simulink model "power_13NodeTestFeeder_4VSC_PV_DEG_symmtrc_loads_"  (R2024b)
settings: Solver=ode15s  StartTime=0.0  StopTime=5  FixedStep=1e-6  MaxStep=1e-4  RelTol=1e-6  AbsTol=1e-8  EnableMultiTasking=on
PreLoadFcn:
  | %power_13NodeTestFeeder_init;
values from neighbouring files (symbols this model uses):
  a = 1.3    [init_para_with_symmtrc_loads.m]
  Cdc = 278e-3    (= 0.278)    [init_para_with_symmtrc_loads.m]
  fg = 60    [a01_scan_VSC_13_feeder.m]    (also in init_para_with_symmtrc_loads.m)
  Gn = 1000    [init_para_with_symmtrc_loads.m]
  H = 8    [init_para_with_symmtrc_loads.m]
  Ipv_n = Isc_n*(Rp+Rs)/Rp    (= 8.21426513558)    [init_para_with_symmtrc_loads.m]
  Isc_n = 8.21    [init_para_with_symmtrc_loads.m]
  k = 1.3806503e-23    [init_para_with_symmtrc_loads.m]    (also in ypm_plot_compare_ana_meas.m = 2)
  Kdroop = Sn/(Rdroop*60)    (= 4166666.66667)    [init_para_with_symmtrc_loads.m]
  KI = 0.0032    [init_para_with_symmtrc_loads.m]
  Ki_C = Rc/tau_C    (= 0.768)    [init_para_with_symmtrc_loads.m]
  Ki_DC = omega_DC^2*Cdc    [init_para_with_symmtrc_loads.m]
  ki_dvpp = kp_dvpp/Ti_dvpp    [init_para_with_symmtrc_loads.m]
  Ki_P = 1/(Ki_pq*tau_P)    [init_para_with_symmtrc_loads.m]
  Ki_PLL = Kp_PLL/tau_PLL    [init_para_with_symmtrc_loads.m]
  Kp_C = Lc/tau_C    (= 0.020372)    [init_para_with_symmtrc_loads.m]
  Kp_DC = 2*xi_DC*omega_DC*Cdc    [init_para_with_symmtrc_loads.m]
  kp_dvpp = -(2*Kdcgain)^-1    [init_para_with_symmtrc_loads.m]
  Kp_P = tau_C/(Ki_pq*tau_P)    [init_para_with_symmtrc_loads.m]
  Kp_PLL = xi_PLL*2*omega_PLL/Vp    [init_para_with_symmtrc_loads.m]
  KV = -0.123    [init_para_with_symmtrc_loads.m]
  kv_Vp = [ 1.021 1.042 1.0174]    [init_para_with_symmtrc_loads.m]
  KVmp = Vmp_n/Voc_n    (= 0.799392097264)    [init_para_with_symmtrc_loads.m]
  Lc = 20.372e-6    (= 2.0372e-05)    [init_para_with_symmtrc_loads.m]
  Lg = Xg /(2*pi*fg)    [init_para_with_symmtrc_loads.m]
  Np = 345    [init_para_with_symmtrc_loads.m]
  Ns = 45    [init_para_with_symmtrc_loads.m]
  Ns_cell = 54    [init_para_with_symmtrc_loads.m]
  p_jump_time = 5    [init_para_with_symmtrc_loads.m]
  p_jump_value = 2*-1e6    (= -2000000)    [init_para_with_symmtrc_loads.m]
  phi_vec = phi_vec_deg/180*pi    [init_para_with_symmtrc_loads.m]
  ppv_nom = 4.9687e+05    (= 496870)    [init_para_with_symmtrc_loads.m]
  q = 1.6021764e-19    [init_para_with_symmtrc_loads.m]
  Rc = 0.768e-3    (= 0.000768)    [init_para_with_symmtrc_loads.m]
  Rg = (U_rms^2 / S_sc) / (sqrt(1 + XoverR^2))    [init_para_with_symmtrc_loads.m]
  Rp = 425.405    [init_para_with_symmtrc_loads.m]
  Rs = 0.221    [init_para_with_symmtrc_loads.m]
  S_base_all = 1    [init_para_with_symmtrc_loads.m]
  Sn = 15e6    (= 15000000)    [init_para_with_symmtrc_loads.m]
  tau_PLL = 2*xi_PLL/omega_PLL    [init_para_with_symmtrc_loads.m]
  Tn = 25    [init_para_with_symmtrc_loads.m]
  Ts = T_ctrl/n_ctrl    [a01_scan_VSC_13_feeder.m]    (also in init_para_with_symmtrc_loads.m = 5e-05)
  U_rms = 4160    [init_para_with_symmtrc_loads.m]
  Vdc = 1200    [init_para_with_symmtrc_loads.m]
  Voc_n = 32.9    [init_para_with_symmtrc_loads.m]
  Vp = sqrt(2)*480/sqrt(3)    [a01_scan_VSC_13_feeder.m]    (also in init_para_with_symmtrc_loads.m = Ug*sqrt(2)/sqrt(3))
undefined symbols (not defined in the file or in its folder): j, Newton, para_grid, para_PVgeno, Raphson
libraries: spsabctoAlphaBetaZeroLib x141, spsPower3phInstantaneousLib x70, spsSeriesRLCBranchLib x44, spsThreePhaseVIMeasurementLib x27, slpidlib x24, spsThreePhaseSeriesRLCLoadLib x15, spsControlledVoltageSourceLib x15, spsMeanLib x9, spsCurrentMeasurementLib x8, spsControlledCurrentSourceLib x8, cstblocks x8, spsGroundLib x5
(part 7 of 10)

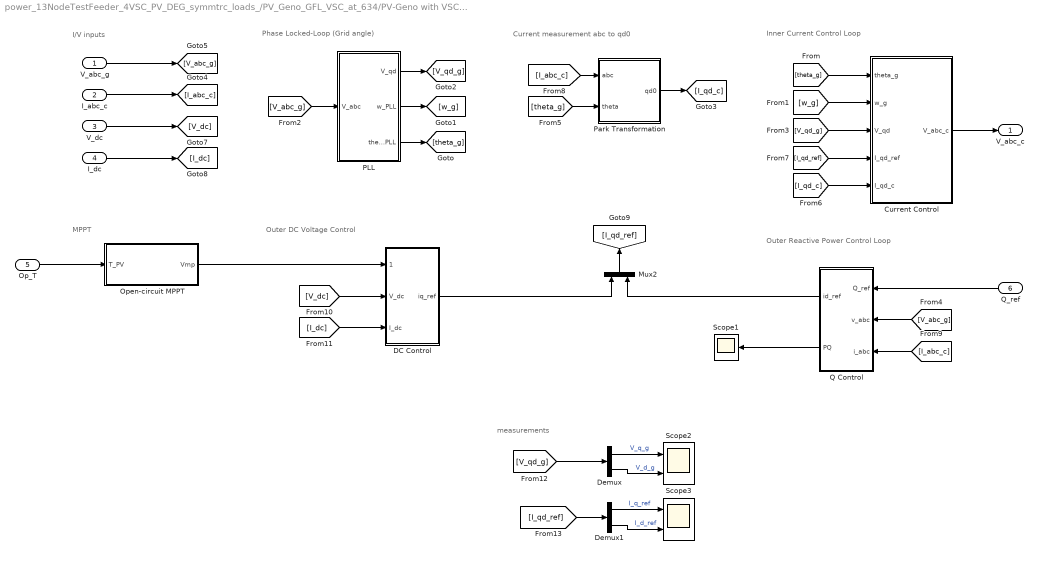
== system power_13NodeTestFeeder_4VSC_PV_DEG_symmtrc_loads_/PV_Geno_GFL_VSC_at_634/PV-Geno with VSC_GFL_at_634     /VSC Control ==
  note: I/V inputs
  note: Phase Locked-Loop (Grid angle)
  note: Current measurement abc to qd0
  note: Inner Current Control Loop
  note: Outer Reactive Power Control Loop
  note: MPPT
  note: Outer DC Voltage Control
  note: measurements
  V_abc_g : Inport
  I_abc_c : Inport  Port=2
  V_dc : Inport  Port=3
  I_dc : Inport  Port=4
  Op_T : Inport  Port=5
  Q_ref : Inport  Port=6
  Current Control : Subsystem
  DC Control : Subsystem
  Demux : Demux  Outputs=2
  Demux1 : Demux  Outputs=2
  Mux2 : Mux  Inputs=2
  Open-circuit MPPT : Subsystem
  PLL : Subsystem
  Park Transformation : Subsystem
  Q Control : Subsystem
  Scope1 : Scope
  Scope2 : Scope  NumInputPorts=2
  Scope3 : Scope  NumInputPorts=2
  V_abc_c : Outport
  wires:
  Park Transformation/1(qd0) -> [I_qd_c]
  [theta_g] -> Current Control/1(theta_g)
  PLL/3(theta_PLL) -> [theta_g]
  [I_qd_ref] -> Current Control/4(I_qd_ref)
  [theta_g] -> Park Transformation/2(theta)
  PLL/1(V_qd) -> [V_qd_g]
  PLL/2(w_PLL) -> [w_g]
  [w_g] -> Current Control/2(w_g)
  [V_qd_g] -> Current Control/3(V_qd)
  [I_qd_c] -> Current Control/5(I_qd_c)
  Current Control/1(V_abc_c) -> V_abc_c/1
  [V_abc_g] -> Q Control/2(v_abc)
  [I_abc_c] -> Q Control/3(i_abc)
  [V_dc] -> DC Control/2(V_dc)
  [I_dc] -> DC Control/3(I_dc)
  [I_abc_c] -> Park Transformation/1(abc)
  V_dc/1 -> [V_dc]
  I_abc_c/1 -> [I_abc_c]
  V_abc_g/1 -> [V_abc_g]
  I_dc/1 -> [I_dc]
  DC Control/1(iq_ref) -> Mux2/1
  Q Control/1(id_ref) -> Mux2/2
  Mux2/1 -> [I_qd_ref]
  Q_ref/1 -> Q Control/1(Q_ref)
  Op_T/1 -> Open-circuit MPPT/1(T_PV)
  Q Control/2(PQ) -> Scope1/1
  Open-circuit MPPT/1(Vmp) -> DC Control/1(V_dc_ref)
  [V_abc_g] -> PLL/1(V_abc)
  Demux/2 -> Scope2/2  "V_d_g"
  Demux1/2 -> Scope3/2  "I_d_ref"
  Demux/1 -> Scope2/1  "V_q_g"
  [V_qd_g] -> Demux/1
  Demux1/1 -> Scope3/1  "I_q_ref"
  [I_qd_ref] -> Demux1/1

== system power_13NodeTestFeeder_4VSC_PV_DEG_symmtrc_loads_/PV_Geno_GFL_VSC_at_672/PV-Geno with VSC_GFL_at_672/PV Array ==
  note: Allows PV model to initialize
  T : Inport
  G : Inport  Port=2
  V_dc : Inport  Port=3
  I_dc : Inport  Port=4
  Controlled Current Source19 : spsControlledCurrentSourceLib/Controlled Current Source  Initialize=on  Source_Type=AC  Amplitude=0  Phase=0  Frequency=0  Measurements=None
  Display : Display
  I module : MATLABFcn  MATLABFcn=Np*u(2)-Np*u(1)*(exp((u(3)/(Ns)+Rs*u(4)/Np)/((Ns_cell*k*(u(5)+273.15)/q)*a))-1)-Np*((u(3)/(Ns)+Rs*u(4)/Np)/Rp)  OutputDimensions=1
  I0 : MATLABFcn  MATLABFcn=(Isc_n+KI*(u(1)-Tn))/(exp((Voc_n+KV*(u(1)-Tn))/((Ns_cell*k*(u(1)+273.15)/q)*a))-1);  OutputDimensions=1
  Ipv : MATLABFcn  MATLABFcn=(Ipv_n+KI*(u(1)-Tn))*(u(2)/Gn);  OutputDimensions=1
  Memory : Memory
  Memory1 : Memory
  Mux : Mux  Inputs=2
  Mux1 : Mux  Inputs=5
  Product17 : Product
  Saturation : Saturate  UpperLimit=10e6  LowerLimit=0.1
  Step16 : Step  Time=0.001  SampleTime=0
  PV+ : PMIOPort  Side=Right
  PV- : PMIOPort  Port=2  Side=Right
  wires:
  Mux1/1 -> I module/1
  G/1 -> Mux/2
  Mux/1 -> Ipv/1
  T/1 -> Mux1/5, Mux/1, I0/1
  Ipv/1 -> Mux1/2
  I0/1 -> Mux1/1
  Memory/1 -> Mux1/4
  I_dc/1 -> Memory/1
  Saturation/1 -> Product17/1
  Step16/1 -> Product17/2
  Product17/1 -> Controlled Current Source19/1
  Memory1/1 -> Mux1/3
  V_dc/1 -> Memory1/1
  I module/1 -> Display/1, Saturation/1
  connections:
  PV+/RConn1 -- Controlled Current Source19/RConn1
  Controlled Current Source19/LConn1 -- PV-/RConn1

== system power_13NodeTestFeeder_4VSC_PV_DEG_symmtrc_loads_/PV_Geno_GFL_VSC_at_672/PV-Geno with VSC_GFL_at_672/VSC ==
  V_abc_c : Inport
  I_abc_c : Inport  Port=2
  V_dc : Inport  Port=3
  Controlled Current Source1 : spsControlledCurrentSourceLib/Controlled Current Source  Initialize=on  Source_Type=AC  Amplitude=0  Phase=0  Frequency=0  Measurements=None
  Controlled Voltage Source3 : spsControlledVoltageSourceLib/Controlled Voltage Source  Initialize=off  Source_Type=AC  Amplitude=0  Phase=0  Frequency=60  Measurements=None
  Controlled Voltage Source4 : spsControlledVoltageSourceLib/Controlled Voltage Source  Initialize=off  Source_Type=AC  Amplitude=0  Phase=0  Frequency=60  Measurements=None
  Controlled Voltage Source5 : spsControlledVoltageSourceLib/Controlled Voltage Source  Initialize=off  Source_Type=AC  Amplitude=0  Phase=0  Frequency=60  Measurements=None
  Delay : Delay  DelayLength=1  InitialCondition=1200
  Demux : Demux  Outputs=3
  Divide : Product  Inputs=*/  RndMeth=Zero  SaturateOnIntegerOverflow=on
  Ground : spsGroundLib/Ground  LConnTagsString=a
  Product : Product
  Sum of Elements : Sum  Inputs=+
  Va_c : PMIOPort  Side=Left
  Vb_c : PMIOPort  Port=2  Side=Left
  Vc_c : PMIOPort  Port=3  Side=Left
  dc+ : PMIOPort  Port=4  Side=Right
  dc- : PMIOPort  Port=5  Side=Right
  wires:
  Product/1 -> Sum of Elements/1
  I_abc_c/1 -> Product/2
  V_abc_c/1 -> Demux/1, Product/1
  Demux/2 -> Controlled Voltage Source4/1
  Demux/1 -> Controlled Voltage Source3/1
  Demux/3 -> Controlled Voltage Source5/1
  Sum of Elements/1 -> Divide/1
  Divide/1 -> Controlled Current Source1/1
  V_dc/1 -> Delay/1
  Delay/1 -> Divide/2
  connections:
  Vb_c/RConn1 -- Controlled Voltage Source4/RConn1
  Va_c/RConn1 -- Controlled Voltage Source3/RConn1
  Controlled Voltage Source4/LConn1 -- Controlled Voltage Source3/LConn1 -- Controlled Voltage Source5/LConn1 -- Ground/LConn1
  Vc_c/RConn1 -- Controlled Voltage Source5/RConn1
  Controlled Current Source1/RConn1 -- dc-/RConn1
  dc+/RConn1 -- Controlled Current Source1/LConn1

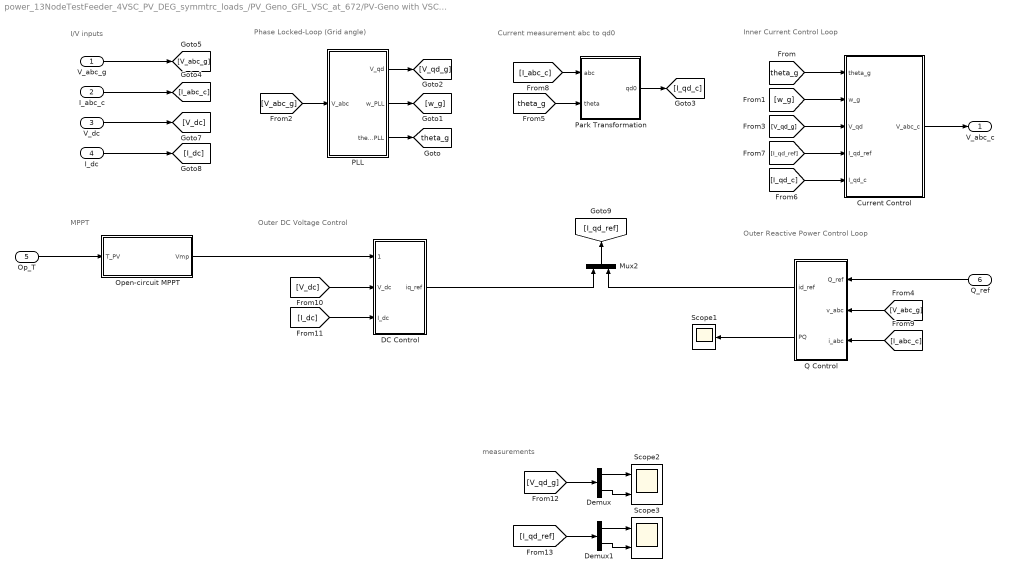
== system power_13NodeTestFeeder_4VSC_PV_DEG_symmtrc_loads_/PV_Geno_GFL_VSC_at_672/PV-Geno with VSC_GFL_at_672/VSC Control ==
  note: I/V inputs
  note: Phase Locked-Loop (Grid angle)
  note: Current measurement abc to qd0
  note: Inner Current Control Loop
  note: Outer Reactive Power Control Loop
  note: MPPT
  note: Outer DC Voltage Control
  note: measurements
  V_abc_g : Inport
  I_abc_c : Inport  Port=2
  V_dc : Inport  Port=3
  I_dc : Inport  Port=4
  Op_T : Inport  Port=5
  Q_ref : Inport  Port=6
  Current Control : Subsystem
  DC Control : Subsystem
  Demux : Demux  Outputs=2
  Demux1 : Demux  Outputs=2
  Mux2 : Mux  Inputs=2
  Open-circuit MPPT : Subsystem
  PLL : Subsystem
  Park Transformation : Subsystem
  Q Control : Subsystem
  Scope1 : Scope
  Scope2 : Scope  NumInputPorts=2
  Scope3 : Scope  NumInputPorts=2
  V_abc_c : Outport
  tag scope: theta_g=global
  wires:
  Park Transformation/1(qd0) -> [I_qd_c]
  [theta_g] -> Current Control/1(theta_g)
  PLL/3(theta_PLL) -> [theta_g]
  [I_qd_ref] -> Current Control/4(I_qd_ref)
  [theta_g] -> Park Transformation/2(theta)
  PLL/1(V_qd) -> [V_qd_g]
  PLL/2(w_PLL) -> [w_g]
  [w_g] -> Current Control/2(w_g)
  [V_qd_g] -> Current Control/3(V_qd)
  [I_qd_c] -> Current Control/5(I_qd_c)
  Current Control/1(V_abc_c) -> V_abc_c/1
  [V_abc_g] -> Q Control/2(v_abc)
  [I_abc_c] -> Q Control/3(i_abc)
  [V_dc] -> DC Control/2(V_dc)
  [I_dc] -> DC Control/3(I_dc)
  [I_abc_c] -> Park Transformation/1(abc)
  V_dc/1 -> [V_dc]
  I_abc_c/1 -> [I_abc_c]
  V_abc_g/1 -> [V_abc_g]
  I_dc/1 -> [I_dc]
  DC Control/1(iq_ref) -> Mux2/1
  Q Control/1(id_ref) -> Mux2/2
  Mux2/1 -> [I_qd_ref]
  Q_ref/1 -> Q Control/1(Q_ref)
  Op_T/1 -> Open-circuit MPPT/1(T_PV)
  Q Control/2(PQ) -> Scope1/1
  Open-circuit MPPT/1(Vmp) -> DC Control/1(V_dc_ref)
  [V_abc_g] -> PLL/1(V_abc)
  Demux/2 -> Scope2/2
  Demux1/2 -> Scope3/2
  Demux/1 -> Scope2/1
  [V_qd_g] -> Demux/1
  Demux1/1 -> Scope3/1
  [I_qd_ref] -> Demux1/1

== system power_13NodeTestFeeder_4VSC_PV_DEG_symmtrc_loads_/PV_Geno_GFL_VSC_at_675/PV-Geno with VSC_GFL_at_675/PV Array ==
  note: Allows PV model to initialize
  T : Inport
  G : Inport  Port=2
  V_dc : Inport  Port=3
  I_dc : Inport  Port=4
  Controlled Current Source19 : spsControlledCurrentSourceLib/Controlled Current Source  Initialize=on  Source_Type=AC  Amplitude=0  Phase=0  Frequency=0  Measurements=None
  Display : Display
  I module : MATLABFcn  MATLABFcn=Np*u(2)-Np*u(1)*(exp((u(3)/(Ns)+Rs*u(4)/Np)/((Ns_cell*k*(u(5)+273.15)/q)*a))-1)-Np*((u(3)/(Ns)+Rs*u(4)/Np)/Rp)  OutputDimensions=1
  I0 : MATLABFcn  MATLABFcn=(Isc_n+KI*(u(1)-Tn))/(exp((Voc_n+KV*(u(1)-Tn))/((Ns_cell*k*(u(1)+273.15)/q)*a))-1);  OutputDimensions=1
  Ipv : MATLABFcn  MATLABFcn=(Ipv_n+KI*(u(1)-Tn))*(u(2)/Gn);  OutputDimensions=1
  Memory : Memory
  Memory1 : Memory
  Mux : Mux  Inputs=2
  Mux1 : Mux  Inputs=5
  Product17 : Product
  Saturation : Saturate  UpperLimit=10e6  LowerLimit=0.1
  Step16 : Step  Time=0.001  SampleTime=0
  PV+ : PMIOPort  Side=Right
  PV- : PMIOPort  Port=2  Side=Right
  wires:
  Mux1/1 -> I module/1
  G/1 -> Mux/2
  Mux/1 -> Ipv/1
  T/1 -> Mux1/5, Mux/1, I0/1
  Ipv/1 -> Mux1/2
  I0/1 -> Mux1/1
  Memory/1 -> Mux1/4
  I_dc/1 -> Memory/1
  Saturation/1 -> Product17/1
  Step16/1 -> Product17/2
  Product17/1 -> Controlled Current Source19/1
  Memory1/1 -> Mux1/3
  V_dc/1 -> Memory1/1
  I module/1 -> Display/1, Saturation/1
  connections:
  PV+/RConn1 -- Controlled Current Source19/RConn1
  Controlled Current Source19/LConn1 -- PV-/RConn1

== system power_13NodeTestFeeder_4VSC_PV_DEG_symmtrc_loads_/PV_Geno_GFL_VSC_at_675/PV-Geno with VSC_GFL_at_675/VSC ==
  V_abc_c : Inport
  I_abc_c : Inport  Port=2
  V_dc : Inport  Port=3
  Controlled Current Source1 : spsControlledCurrentSourceLib/Controlled Current Source  Initialize=on  Source_Type=AC  Amplitude=0  Phase=0  Frequency=0  Measurements=None
  Controlled Voltage Source3 : spsControlledVoltageSourceLib/Controlled Voltage Source  Initialize=off  Source_Type=AC  Amplitude=0  Phase=0  Frequency=60  Measurements=None
  Controlled Voltage Source4 : spsControlledVoltageSourceLib/Controlled Voltage Source  Initialize=off  Source_Type=AC  Amplitude=0  Phase=0  Frequency=60  Measurements=None
  Controlled Voltage Source5 : spsControlledVoltageSourceLib/Controlled Voltage Source  Initialize=off  Source_Type=AC  Amplitude=0  Phase=0  Frequency=60  Measurements=None
  Delay : Delay  DelayLength=1  InitialCondition=1200
  Demux : Demux  Outputs=3
  Divide : Product  Inputs=*/  RndMeth=Zero  SaturateOnIntegerOverflow=on
  Ground : spsGroundLib/Ground  LConnTagsString=a
  Product : Product
  Sum of Elements : Sum  Inputs=+
  Va_c : PMIOPort  Side=Left
  Vb_c : PMIOPort  Port=2  Side=Left
  Vc_c : PMIOPort  Port=3  Side=Left
  dc+ : PMIOPort  Port=4  Side=Right
  dc- : PMIOPort  Port=5  Side=Right
  wires:
  Product/1 -> Sum of Elements/1
  I_abc_c/1 -> Product/2
  V_abc_c/1 -> Demux/1, Product/1
  Demux/2 -> Controlled Voltage Source4/1
  Demux/1 -> Controlled Voltage Source3/1
  Demux/3 -> Controlled Voltage Source5/1
  Sum of Elements/1 -> Divide/1
  Divide/1 -> Controlled Current Source1/1
  V_dc/1 -> Delay/1
  Delay/1 -> Divide/2
  connections:
  Vb_c/RConn1 -- Controlled Voltage Source4/RConn1
  Va_c/RConn1 -- Controlled Voltage Source3/RConn1
  Controlled Voltage Source4/LConn1 -- Controlled Voltage Source3/LConn1 -- Controlled Voltage Source5/LConn1 -- Ground/LConn1
  Vc_c/RConn1 -- Controlled Voltage Source5/RConn1
  Controlled Current Source1/RConn1 -- dc-/RConn1
  dc+/RConn1 -- Controlled Current Source1/LConn1

== system power_13NodeTestFeeder_4VSC_PV_DEG_symmtrc_loads_/PV_Geno_GFL_VSC_at_675/PV-Geno with VSC_GFL_at_675/VSC Control ==
  note: I/V inputs
  note: Phase Locked-Loop (Grid angle)
  note: Current measurement abc to qd0
  note: Inner Current Control Loop
  note: Outer Reactive Power Control Loop
  note: MPPT
  note: Outer DC Voltage Control
  V_abc_g : Inport
  I_abc_c : Inport  Port=2
  V_dc : Inport  Port=3
  I_dc : Inport  Port=4
  Op_T : Inport  Port=5
  Q_ref : Inport  Port=6
  Current Control : Subsystem
  DC Control : Subsystem
  Mux2 : Mux  Inputs=2
  Open-circuit MPPT : Subsystem
  PLL : Subsystem
  Park Transformation : Subsystem
  Q Control : Subsystem
  Scope1 : Scope
  V_abc_c : Outport
  wires:
  Park Transformation/1(qd0) -> [I_qd_c]
  [theta_g] -> Current Control/1(theta_g)
  PLL/3(theta_PLL) -> [theta_g]
  [I_qd_ref] -> Current Control/4(I_qd_ref)
  [theta_g] -> Park Transformation/2(theta)
  PLL/1(V_qd) -> [V_qd_g]
  PLL/2(w_PLL) -> [w_g]
  [w_g] -> Current Control/2(w_g)
  [V_qd_g] -> Current Control/3(V_qd)
  [I_qd_c] -> Current Control/5(I_qd_c)
  Current Control/1(V_abc_c) -> V_abc_c/1
  [V_abc_g] -> Q Control/2(v_abc)
  [I_abc_c] -> Q Control/3(i_abc)
  [V_dc] -> DC Control/2(V_dc)
  [I_dc] -> DC Control/3(I_dc)
  [I_abc_c] -> Park Transformation/1(abc)
  V_dc/1 -> [V_dc]
  I_abc_c/1 -> [I_abc_c]
  V_abc_g/1 -> [V_abc_g]
  I_dc/1 -> [I_dc]
  DC Control/1(iq_ref) -> Mux2/1
  Q Control/1(id_ref) -> Mux2/2
  Mux2/1 -> [I_qd_ref]
  Q_ref/1 -> Q Control/1(Q_ref)
  Op_T/1 -> Open-circuit MPPT/1(T_PV)
  Q Control/2(PQ) -> Scope1/1
  Open-circuit MPPT/1(Vmp) -> DC Control/1(V_dc_ref)
  [V_abc_g] -> PLL/1(V_abc)

== system power_13NodeTestFeeder_4VSC_PV_DEG_symmtrc_loads_/PV_Geno_GFL_VSC_at_680/PV-Geno with VSC_GFL_at_680/PV Array ==
  note: Allows PV model to initialize
  T : Inport
  G : Inport  Port=2
  V_dc : Inport  Port=3
  I_dc : Inport  Port=4
  Controlled Current Source19 : spsControlledCurrentSourceLib/Controlled Current Source  Initialize=on  Source_Type=AC  Amplitude=0  Phase=0  Frequency=0  Measurements=None
  Display : Display
  I module : MATLABFcn  MATLABFcn=Np*u(2)-Np*u(1)*(exp((u(3)/(Ns)+Rs*u(4)/Np)/((Ns_cell*k*(u(5)+273.15)/q)*a))-1)-Np*((u(3)/(Ns)+Rs*u(4)/Np)/Rp)  OutputDimensions=1
  I0 : MATLABFcn  MATLABFcn=(Isc_n+KI*(u(1)-Tn))/(exp((Voc_n+KV*(u(1)-Tn))/((Ns_cell*k*(u(1)+273.15)/q)*a))-1);  OutputDimensions=1
  Ipv : MATLABFcn  MATLABFcn=(Ipv_n+KI*(u(1)-Tn))*(u(2)/Gn);  OutputDimensions=1
  Memory : Memory
  Memory1 : Memory
  Mux : Mux  Inputs=2
  Mux1 : Mux  Inputs=5
  Product17 : Product
  Saturation : Saturate  UpperLimit=10e6  LowerLimit=0.1
  Step16 : Step  Time=0.001  SampleTime=0
  PV+ : PMIOPort  Side=Right
  PV- : PMIOPort  Port=2  Side=Right
  wires:
  I module/1 -> Saturation/1, Display/1
  V_dc/1 -> Memory1/1
  Memory1/1 -> Mux1/3
  Product17/1 -> Controlled Current Source19/1
  Step16/1 -> Product17/2
  Saturation/1 -> Product17/1
  I_dc/1 -> Memory/1
  Memory/1 -> Mux1/4
  I0/1 -> Mux1/1
  Ipv/1 -> Mux1/2
  T/1 -> I0/1, Mux/1, Mux1/5
  Mux/1 -> Ipv/1
  G/1 -> Mux/2
  Mux1/1 -> I module/1
  connections:
  Controlled Current Source19/LConn1 -- PV-/RConn1
  PV+/RConn1 -- Controlled Current Source19/RConn1

== system power_13NodeTestFeeder_4VSC_PV_DEG_symmtrc_loads_/PV_Geno_GFL_VSC_at_680/PV-Geno with VSC_GFL_at_680/VSC ==
  V_abc_c : Inport
  I_abc_c : Inport  Port=2
  V_dc : Inport  Port=3
  Controlled Current Source1 : spsControlledCurrentSourceLib/Controlled Current Source  Initialize=on  Source_Type=AC  Amplitude=0  Phase=0  Frequency=0  Measurements=None
  Controlled Voltage Source3 : spsControlledVoltageSourceLib/Controlled Voltage Source  Initialize=off  Source_Type=AC  Amplitude=0  Phase=0  Frequency=60  Measurements=None
  Controlled Voltage Source4 : spsControlledVoltageSourceLib/Controlled Voltage Source  Initialize=off  Source_Type=AC  Amplitude=0  Phase=0  Frequency=60  Measurements=None
  Controlled Voltage Source5 : spsControlledVoltageSourceLib/Controlled Voltage Source  Initialize=off  Source_Type=AC  Amplitude=0  Phase=0  Frequency=60  Measurements=None
  Delay : Delay  DelayLength=1  InitialCondition=1200
  Demux : Demux  Outputs=3
  Divide : Product  Inputs=*/  RndMeth=Zero  SaturateOnIntegerOverflow=on
  Ground : spsGroundLib/Ground  LConnTagsString=a
  Product : Product
  Sum of Elements : Sum  Inputs=+
  Va_c : PMIOPort  Side=Left
  Vb_c : PMIOPort  Port=2  Side=Left
  Vc_c : PMIOPort  Port=3  Side=Left
  dc+ : PMIOPort  Port=4  Side=Right
  dc- : PMIOPort  Port=5  Side=Right
  wires:
  Delay/1 -> Divide/2
  V_dc/1 -> Delay/1
  Divide/1 -> Controlled Current Source1/1
  Sum of Elements/1 -> Divide/1
  Demux/3 -> Controlled Voltage Source5/1
  Demux/1 -> Controlled Voltage Source3/1
  Demux/2 -> Controlled Voltage Source4/1
  V_abc_c/1 -> Product/1, Demux/1
  I_abc_c/1 -> Product/2
  Product/1 -> Sum of Elements/1
  connections:
  dc+/RConn1 -- Controlled Current Source1/LConn1
  Controlled Current Source1/RConn1 -- dc-/RConn1
  Vc_c/RConn1 -- Controlled Voltage Source5/RConn1
  Ground/LConn1 -- Controlled Voltage Source5/LConn1 -- Controlled Voltage Source3/LConn1 -- Controlled Voltage Source4/LConn1
  Va_c/RConn1 -- Controlled Voltage Source3/RConn1
  Vb_c/RConn1 -- Controlled Voltage Source4/RConn1

== system power_13NodeTestFeeder_4VSC_PV_DEG_symmtrc_loads_/PV_Geno_GFL_VSC_at_680/PV-Geno with VSC_GFL_at_680/VSC Control ==
  note: measurements
  note: MPPT
  note: Outer Reactive Power Control Loop
  note: Inner Current Control Loop
  note: Current measurement abc to qd0
  note: Phase Locked-Loop (Grid angle)
  note: I/V inputs
  note: Outer DC Voltage Control
  V_abc_g : Inport
  I_abc_c : Inport  Port=2
  V_dc : Inport  Port=3
  I_dc : Inport  Port=4
  Op_T : Inport  Port=5
  Q_ref : Inport  Port=6
  Current Control : Subsystem
  DC Control : Subsystem
  Demux : Demux  Outputs=2
  Demux1 : Demux  Outputs=2
  Mux2 : Mux  Inputs=2
  Open-circuit MPPT : Subsystem
  PLL : Subsystem
  Park Transformation : Subsystem
  Q Control : Subsystem
  Scope1 : Scope
  Scope2 : Scope  NumInputPorts=2
  Scope3 : Scope  NumInputPorts=2
  V_abc_c : Outport
  wires:
  [V_abc_g] -> PLL/1(V_abc)
  Open-circuit MPPT/1(Vmp) -> DC Control/1(V_dc_ref)
  Q Control/2(PQ) -> Scope1/1
  Op_T/1 -> Open-circuit MPPT/1(T_PV)
  Q_ref/1 -> Q Control/1(Q_ref)
  Mux2/1 -> [I_qd_ref]
  Q Control/1(id_ref) -> Mux2/2
  DC Control/1(iq_ref) -> Mux2/1
  I_dc/1 -> [I_dc]
  V_abc_g/1 -> [V_abc_g]
  I_abc_c/1 -> [I_abc_c]
  V_dc/1 -> [V_dc]
  [I_abc_c] -> Park Transformation/1(abc)
  [I_dc] -> DC Control/3(I_dc)
  [V_dc] -> DC Control/2(V_dc)
  [I_abc_c] -> Q Control/3(i_abc)
  [V_abc_g] -> Q Control/2(v_abc)
  Current Control/1(V_abc_c) -> V_abc_c/1
  [I_qd_c] -> Current Control/5(I_qd_c)
  [V_qd_g] -> Current Control/3(V_qd)
  [w_g] -> Current Control/2(w_g)
  PLL/2(w_PLL) -> [w_g]
  PLL/1(V_qd) -> [V_qd_g]
  [theta_g] -> Park Transformation/2(theta)
  [I_qd_ref] -> Current Control/4(I_qd_ref)
  PLL/3(theta_PLL) -> [theta_g]
  [theta_g] -> Current Control/1(theta_g)
  Park Transformation/1(qd0) -> [I_qd_c]
  [V_qd_g] -> Demux/1
  Demux/1 -> Scope2/1
  Demux/2 -> Scope2/2
  Demux1/2 -> Scope3/2
  Demux1/1 -> Scope3/1
  [I_qd_ref] -> Demux1/1

== system power_13NodeTestFeeder_4VSC_PV_DEG_symmtrc_loads_/RMS and Pos // Neg Sequence Calculation /Subsystem/PLL aligned with positive-sequence ==
  note: PLL
      | aligned with vd+
  Vabc : Inport
  0-vd=-vd : Gain  Gain=-1
  Gain : Gain  Gain=1/(2*pi)
  Integrator : Integrator  InitialCondition=pi
  Phase-sequence separation : Subsystem
  Subsystem : Subsystem
      mask Display: disp('PI\n')
  Terminator : Terminator
  Terminator1 : Terminator
  Terminator2 : Terminator
  theta : Outport
  f : Outport  Port=2
  wires:
  Integrator/1 -> theta/1, Phase-sequence separation/2(Theta)
  Gain/1 -> f/1
  0-vd=-vd/1 -> Subsystem/1(in)
  Subsystem/1(w) -> Gain/1, Integrator/1
  Vabc/1 -> Phase-sequence separation/1(abc)
  Phase-sequence separation/1(q+) -> Terminator/1
  Phase-sequence separation/2(d+) -> 0-vd=-vd/1  "vd+"
  Phase-sequence separation/3(q-) -> Terminator1/1
  Phase-sequence separation/4(d-) -> Terminator2/1

== system power_13NodeTestFeeder_4VSC_PV_DEG_symmtrc_loads_/RMS and Pos // Neg Sequence Calculation /Subsystem/Phase-sequence separation1 ==
  note: Phase-sequence separation based on
      | Delayed Signal Cancellation (DSC) method
  abc : Inport
  Theta : Inport  Port=2
  Complex to Real-Imag1 : ComplexToRealImag
  Complex to Real-Imag2 : ComplexToRealImag
  Complex to Real-Imag3 : ComplexToRealImag
  Constant : Constant
  Demux3 : Demux  Outputs=3
  Exp2 : Math  OutputSignalType=complex
  Exp3 : Math  OutputSignalType=complex
  Gain1 : Gain  Gain=1/2
  Gain4 : Gain  Gain=-1i
  Gain5 : Gain  Gain=1i
  Gain6 : Gain  Gain=1/2
  Gain7 : Gain  Gain=1i
  NOT : Logic  Operator=NOT  IconShape=distinctive  AllPortsSameDT=off  OutDataTypeStr=boolean
  Product3 : Product
  Product4 : Product
  Real-Imag to Complex : RealImagToComplex
  Real-Imag to Complex1 : RealImagToComplex
  Sum1 : Sum  Inputs=|++
  Sum2 : Sum  Inputs=-+|
  Switch : Switch  Criteria=u2 ~= 0  SaturateOnIntegerOverflow=off  InputSameDT=off
  Terminator3 : Terminator
  Transport Delay2 : TransportDelay  DelayTime=1/4*(1/fg)  BufferSize=1024*4
  Transport Delay3 : TransportDelay  DelayTime=1/4*(1/fg)  BufferSize=1024*4
  abc to Alpha-Beta-Zero : spsabctoAlphaBetaZeroLib/abc to Alpha-Beta-Zero
  q+ : Outport
  d+ : Outport  Port=2
  q- : Outport  Port=3
  d- : Outport  Port=4
  wires:
  NOT/1 -> Switch/2
  Constant/1 -> NOT/1
  Switch/1 -> Product3/1
  Gain6/1 -> Switch/3
  Sum2/1 -> Gain1/1
  Transport Delay2/1 -> Real-Imag to Complex1/1
  Demux3/1 -> Real-Imag to Complex/1
  Complex to Real-Imag1/2 -> Transport Delay3/1
  Gain1/1 -> Product4/2
  Real-Imag to Complex/1 -> Complex to Real-Imag1/1, Sum2/2, Sum1/1, Switch/1
  Complex to Real-Imag3/1 -> d-/1
  Real-Imag to Complex1/1 -> Gain5/1
  Complex to Real-Imag1/1 -> Transport Delay2/1
  Transport Delay3/1 -> Real-Imag to Complex1/2
  Demux3/2 -> Real-Imag to Complex/2
  Product3/1 -> Complex to Real-Imag2/1
  Product4/1 -> Complex to Real-Imag3/1
  abc to Alpha-Beta-Zero/1 -> Demux3/1
  abc/1 -> abc to Alpha-Beta-Zero/1
  Exp3/1 -> Product4/1
  Complex to Real-Imag3/2 -> q-/1
  Complex to Real-Imag2/2 -> q+/1
  Demux3/3 -> Terminator3/1
  Sum1/1 -> Gain6/1
  Gain5/1 -> Sum2/1, Sum1/2
  Exp2/1 -> Product3/2
  Gain4/1 -> Exp2/1
  Theta/1 -> Gain4/1, Gain7/1
  Gain7/1 -> Exp3/1
  Complex to Real-Imag2/1 -> d+/1

== system power_13NodeTestFeeder_4VSC_PV_DEG_symmtrc_loads_/RMS and Pos // Neg Sequence Calculation /Subsystem/Phase-sequence separation2 ==
  note: Phase-sequence separation based on
      | Delayed Signal Cancellation (DSC) method
  abc : Inport
  Theta : Inport  Port=2
  Complex to Real-Imag1 : ComplexToRealImag
  Complex to Real-Imag2 : ComplexToRealImag
  Complex to Real-Imag3 : ComplexToRealImag
  Constant : Constant
  Demux3 : Demux  Outputs=3
  Exp2 : Math  OutputSignalType=complex
  Exp3 : Math  OutputSignalType=complex
  Gain1 : Gain  Gain=1/2
  Gain4 : Gain  Gain=-1i
  Gain5 : Gain  Gain=1i
  Gain6 : Gain  Gain=1/2
  Gain7 : Gain  Gain=1i
  NOT : Logic  Operator=NOT  IconShape=distinctive  AllPortsSameDT=off  OutDataTypeStr=boolean
  Product3 : Product
  Product4 : Product
  Real-Imag to Complex : RealImagToComplex
  Real-Imag to Complex1 : RealImagToComplex
  Sum1 : Sum  Inputs=|++
  Sum2 : Sum  Inputs=-+|
  Switch : Switch  Criteria=u2 ~= 0  SaturateOnIntegerOverflow=off  InputSameDT=off
  Terminator3 : Terminator
  Transport Delay2 : TransportDelay  DelayTime=1/4*(1/fg)  BufferSize=1024*4
  Transport Delay3 : TransportDelay  DelayTime=1/4*(1/fg)  BufferSize=1024*4
  abc to Alpha-Beta-Zero : spsabctoAlphaBetaZeroLib/abc to Alpha-Beta-Zero
  q+ : Outport
  d+ : Outport  Port=2
  q- : Outport  Port=3
  d- : Outport  Port=4
  wires:
  NOT/1 -> Switch/2
  Constant/1 -> NOT/1
  Switch/1 -> Product3/1
  Gain6/1 -> Switch/3
  Sum2/1 -> Gain1/1
  Transport Delay2/1 -> Real-Imag to Complex1/1
  Demux3/1 -> Real-Imag to Complex/1
  Complex to Real-Imag1/2 -> Transport Delay3/1
  Gain1/1 -> Product4/2
  Real-Imag to Complex/1 -> Complex to Real-Imag1/1, Sum2/2, Sum1/1, Switch/1
  Complex to Real-Imag3/1 -> d-/1
  Real-Imag to Complex1/1 -> Gain5/1
  Complex to Real-Imag1/1 -> Transport Delay2/1
  Transport Delay3/1 -> Real-Imag to Complex1/2
  Demux3/2 -> Real-Imag to Complex/2
  Product3/1 -> Complex to Real-Imag2/1
  Product4/1 -> Complex to Real-Imag3/1
  abc to Alpha-Beta-Zero/1 -> Demux3/1
  abc/1 -> abc to Alpha-Beta-Zero/1
  Exp3/1 -> Product4/1
  Complex to Real-Imag3/2 -> q-/1
  Complex to Real-Imag2/2 -> q+/1
  Demux3/3 -> Terminator3/1
  Sum1/1 -> Gain6/1
  Gain5/1 -> Sum2/1, Sum1/2
  Exp2/1 -> Product3/2
  Gain4/1 -> Exp2/1
  Theta/1 -> Gain4/1, Gain7/1
  Gain7/1 -> Exp3/1
  Complex to Real-Imag2/1 -> d+/1

== system power_13NodeTestFeeder_4VSC_PV_DEG_symmtrc_loads_/RMS and Pos // Neg Sequence Calculation /Subsystem1/PLL aligned with positive-sequence ==
  note: PLL
      | aligned with vd+
  Vabc : Inport
  0-vd=-vd : Gain  Gain=-1
  Gain : Gain  Gain=1/(2*pi)
  Integrator : Integrator  InitialCondition=pi
  Phase-sequence separation : Subsystem
  Subsystem : Subsystem
      mask Display: disp('PI\n')
  Terminator : Terminator
  Terminator1 : Terminator
  Terminator2 : Terminator
  theta : Outport
  f : Outport  Port=2
  wires:
  Integrator/1 -> theta/1, Phase-sequence separation/2(Theta)
  Gain/1 -> f/1
  0-vd=-vd/1 -> Subsystem/1(in)
  Subsystem/1(w) -> Gain/1, Integrator/1
  Vabc/1 -> Phase-sequence separation/1(abc)
  Phase-sequence separation/1(q+) -> Terminator/1
  Phase-sequence separation/2(d+) -> 0-vd=-vd/1  "vd+"
  Phase-sequence separation/3(q-) -> Terminator1/1
  Phase-sequence separation/4(d-) -> Terminator2/1

== system power_13NodeTestFeeder_4VSC_PV_DEG_symmtrc_loads_/RMS and Pos // Neg Sequence Calculation /Subsystem1/Phase-sequence separation1 ==
  note: Phase-sequence separation based on
      | Delayed Signal Cancellation (DSC) method
  abc : Inport
  Theta : Inport  Port=2
  Complex to Real-Imag1 : ComplexToRealImag
  Complex to Real-Imag2 : ComplexToRealImag
  Complex to Real-Imag3 : ComplexToRealImag
  Constant : Constant
  Demux3 : Demux  Outputs=3
  Exp2 : Math  OutputSignalType=complex
  Exp3 : Math  OutputSignalType=complex
  Gain1 : Gain  Gain=1/2
  Gain4 : Gain  Gain=-1i
  Gain5 : Gain  Gain=1i
  Gain6 : Gain  Gain=1/2
  Gain7 : Gain  Gain=1i
  NOT : Logic  Operator=NOT  IconShape=distinctive  AllPortsSameDT=off  OutDataTypeStr=boolean
  Product3 : Product
  Product4 : Product
  Real-Imag to Complex : RealImagToComplex
  Real-Imag to Complex1 : RealImagToComplex
  Sum1 : Sum  Inputs=|++
  Sum2 : Sum  Inputs=-+|
  Switch : Switch  Criteria=u2 ~= 0  SaturateOnIntegerOverflow=off  InputSameDT=off
  Terminator3 : Terminator
  Transport Delay2 : TransportDelay  DelayTime=1/4*(1/fg)  BufferSize=1024*4
  Transport Delay3 : TransportDelay  DelayTime=1/4*(1/fg)  BufferSize=1024*4
  abc to Alpha-Beta-Zero : spsabctoAlphaBetaZeroLib/abc to Alpha-Beta-Zero
  q+ : Outport
  d+ : Outport  Port=2
  q- : Outport  Port=3
  d- : Outport  Port=4
  wires:
  NOT/1 -> Switch/2
  Constant/1 -> NOT/1
  Switch/1 -> Product3/1
  Gain6/1 -> Switch/3
  Sum2/1 -> Gain1/1
  Transport Delay2/1 -> Real-Imag to Complex1/1
  Demux3/1 -> Real-Imag to Complex/1
  Complex to Real-Imag1/2 -> Transport Delay3/1
  Gain1/1 -> Product4/2
  Real-Imag to Complex/1 -> Complex to Real-Imag1/1, Sum2/2, Sum1/1, Switch/1
  Complex to Real-Imag3/1 -> d-/1
  Real-Imag to Complex1/1 -> Gain5/1
  Complex to Real-Imag1/1 -> Transport Delay2/1
  Transport Delay3/1 -> Real-Imag to Complex1/2
  Demux3/2 -> Real-Imag to Complex/2
  Product3/1 -> Complex to Real-Imag2/1
  Product4/1 -> Complex to Real-Imag3/1
  abc to Alpha-Beta-Zero/1 -> Demux3/1
  abc/1 -> abc to Alpha-Beta-Zero/1
  Exp3/1 -> Product4/1
  Complex to Real-Imag3/2 -> q-/1
  Complex to Real-Imag2/2 -> q+/1
  Demux3/3 -> Terminator3/1
  Sum1/1 -> Gain6/1
  Gain5/1 -> Sum2/1, Sum1/2
  Exp2/1 -> Product3/2
  Gain4/1 -> Exp2/1
  Theta/1 -> Gain4/1, Gain7/1
  Gain7/1 -> Exp3/1
  Complex to Real-Imag2/1 -> d+/1

== system power_13NodeTestFeeder_4VSC_PV_DEG_symmtrc_loads_/RMS and Pos // Neg Sequence Calculation /Subsystem1/Phase-sequence separation2 ==
  note: Phase-sequence separation based on
      | Delayed Signal Cancellation (DSC) method
  abc : Inport
  Theta : Inport  Port=2
  Complex to Real-Imag1 : ComplexToRealImag
  Complex to Real-Imag2 : ComplexToRealImag
  Complex to Real-Imag3 : ComplexToRealImag
  Constant : Constant
  Demux3 : Demux  Outputs=3
  Exp2 : Math  OutputSignalType=complex
  Exp3 : Math  OutputSignalType=complex
  Gain1 : Gain  Gain=1/2
  Gain4 : Gain  Gain=-1i
  Gain5 : Gain  Gain=1i
  Gain6 : Gain  Gain=1/2
  Gain7 : Gain  Gain=1i
  NOT : Logic  Operator=NOT  IconShape=distinctive  AllPortsSameDT=off  OutDataTypeStr=boolean
  Product3 : Product
  Product4 : Product
  Real-Imag to Complex : RealImagToComplex
  Real-Imag to Complex1 : RealImagToComplex
  Sum1 : Sum  Inputs=|++
  Sum2 : Sum  Inputs=-+|
  Switch : Switch  Criteria=u2 ~= 0  SaturateOnIntegerOverflow=off  InputSameDT=off
  Terminator3 : Terminator
  Transport Delay2 : TransportDelay  DelayTime=1/4*(1/fg)  BufferSize=1024*4
  Transport Delay3 : TransportDelay  DelayTime=1/4*(1/fg)  BufferSize=1024*4
  abc to Alpha-Beta-Zero : spsabctoAlphaBetaZeroLib/abc to Alpha-Beta-Zero
  q+ : Outport
  d+ : Outport  Port=2
  q- : Outport  Port=3
  d- : Outport  Port=4
  wires:
  NOT/1 -> Switch/2
  Constant/1 -> NOT/1
  Switch/1 -> Product3/1
  Gain6/1 -> Switch/3
  Sum2/1 -> Gain1/1
  Transport Delay2/1 -> Real-Imag to Complex1/1
  Demux3/1 -> Real-Imag to Complex/1
  Complex to Real-Imag1/2 -> Transport Delay3/1
  Gain1/1 -> Product4/2
  Real-Imag to Complex/1 -> Complex to Real-Imag1/1, Sum2/2, Sum1/1, Switch/1
  Complex to Real-Imag3/1 -> d-/1
  Real-Imag to Complex1/1 -> Gain5/1
  Complex to Real-Imag1/1 -> Transport Delay2/1
  Transport Delay3/1 -> Real-Imag to Complex1/2
  Demux3/2 -> Real-Imag to Complex/2
  Product3/1 -> Complex to Real-Imag2/1
  Product4/1 -> Complex to Real-Imag3/1
  abc to Alpha-Beta-Zero/1 -> Demux3/1
  abc/1 -> abc to Alpha-Beta-Zero/1
  Exp3/1 -> Product4/1
  Complex to Real-Imag3/2 -> q-/1
  Complex to Real-Imag2/2 -> q+/1
  Demux3/3 -> Terminator3/1
  Sum1/1 -> Gain6/1
  Gain5/1 -> Sum2/1, Sum1/2
  Exp2/1 -> Product3/2
  Gain4/1 -> Exp2/1
  Theta/1 -> Gain4/1, Gain7/1
  Gain7/1 -> Exp3/1
  Complex to Real-Imag2/1 -> d+/1

== system power_13NodeTestFeeder_4VSC_PV_DEG_symmtrc_loads_/RMS and Pos // Neg Sequence Calculation /Subsystem2/PLL aligned with positive-sequence ==
  note: PLL
      | aligned with vd+
  Vabc : Inport
  0-vd=-vd : Gain  Gain=-1
  Gain : Gain  Gain=1/(2*pi)
  Integrator : Integrator  InitialCondition=pi
  Phase-sequence separation : Subsystem
  Subsystem : Subsystem
      mask Display: disp('PI\n')
  Terminator : Terminator
  Terminator1 : Terminator
  Terminator2 : Terminator
  theta : Outport
  f : Outport  Port=2
  wires:
  Integrator/1 -> theta/1, Phase-sequence separation/2(Theta)
  Gain/1 -> f/1
  0-vd=-vd/1 -> Subsystem/1(in)
  Subsystem/1(w) -> Gain/1, Integrator/1
  Vabc/1 -> Phase-sequence separation/1(abc)
  Phase-sequence separation/1(q+) -> Terminator/1
  Phase-sequence separation/2(d+) -> 0-vd=-vd/1  "vd+"
  Phase-sequence separation/3(q-) -> Terminator1/1
  Phase-sequence separation/4(d-) -> Terminator2/1

== system power_13NodeTestFeeder_4VSC_PV_DEG_symmtrc_loads_/RMS and Pos // Neg Sequence Calculation /Subsystem2/Phase-sequence separation1 ==
  note: Phase-sequence separation based on
      | Delayed Signal Cancellation (DSC) method
  abc : Inport
  Theta : Inport  Port=2
  Complex to Real-Imag1 : ComplexToRealImag
  Complex to Real-Imag2 : ComplexToRealImag
  Complex to Real-Imag3 : ComplexToRealImag
  Constant : Constant
  Demux3 : Demux  Outputs=3
  Exp2 : Math  OutputSignalType=complex
  Exp3 : Math  OutputSignalType=complex
  Gain1 : Gain  Gain=1/2
  Gain4 : Gain  Gain=-1i
  Gain5 : Gain  Gain=1i
  Gain6 : Gain  Gain=1/2
  Gain7 : Gain  Gain=1i
  NOT : Logic  Operator=NOT  IconShape=distinctive  AllPortsSameDT=off  OutDataTypeStr=boolean
  Product3 : Product
  Product4 : Product
  Real-Imag to Complex : RealImagToComplex
  Real-Imag to Complex1 : RealImagToComplex
  Sum1 : Sum  Inputs=|++
  Sum2 : Sum  Inputs=-+|
  Switch : Switch  Criteria=u2 ~= 0  SaturateOnIntegerOverflow=off  InputSameDT=off
  Terminator3 : Terminator
  Transport Delay2 : TransportDelay  DelayTime=1/4*(1/fg)  BufferSize=1024*4
  Transport Delay3 : TransportDelay  DelayTime=1/4*(1/fg)  BufferSize=1024*4
  abc to Alpha-Beta-Zero : spsabctoAlphaBetaZeroLib/abc to Alpha-Beta-Zero
  q+ : Outport
  d+ : Outport  Port=2
  q- : Outport  Port=3
  d- : Outport  Port=4
  wires:
  NOT/1 -> Switch/2
  Constant/1 -> NOT/1
  Switch/1 -> Product3/1
  Gain6/1 -> Switch/3
  Sum2/1 -> Gain1/1
  Transport Delay2/1 -> Real-Imag to Complex1/1
  Demux3/1 -> Real-Imag to Complex/1
  Complex to Real-Imag1/2 -> Transport Delay3/1
  Gain1/1 -> Product4/2
  Real-Imag to Complex/1 -> Complex to Real-Imag1/1, Sum2/2, Sum1/1, Switch/1
  Complex to Real-Imag3/1 -> d-/1
  Real-Imag to Complex1/1 -> Gain5/1
  Complex to Real-Imag1/1 -> Transport Delay2/1
  Transport Delay3/1 -> Real-Imag to Complex1/2
  Demux3/2 -> Real-Imag to Complex/2
  Product3/1 -> Complex to Real-Imag2/1
  Product4/1 -> Complex to Real-Imag3/1
  abc to Alpha-Beta-Zero/1 -> Demux3/1
  abc/1 -> abc to Alpha-Beta-Zero/1
  Exp3/1 -> Product4/1
  Complex to Real-Imag3/2 -> q-/1
  Complex to Real-Imag2/2 -> q+/1
  Demux3/3 -> Terminator3/1
  Sum1/1 -> Gain6/1
  Gain5/1 -> Sum2/1, Sum1/2
  Exp2/1 -> Product3/2
  Gain4/1 -> Exp2/1
  Theta/1 -> Gain4/1, Gain7/1
  Gain7/1 -> Exp3/1
  Complex to Real-Imag2/1 -> d+/1

== system power_13NodeTestFeeder_4VSC_PV_DEG_symmtrc_loads_/RMS and Pos // Neg Sequence Calculation /Subsystem2/Phase-sequence separation2 ==
  note: Phase-sequence separation based on
      | Delayed Signal Cancellation (DSC) method
  abc : Inport
  Theta : Inport  Port=2
  Complex to Real-Imag1 : ComplexToRealImag
  Complex to Real-Imag2 : ComplexToRealImag
  Complex to Real-Imag3 : ComplexToRealImag
  Constant : Constant
  Demux3 : Demux  Outputs=3
  Exp2 : Math  OutputSignalType=complex
  Exp3 : Math  OutputSignalType=complex
  Gain1 : Gain  Gain=1/2
  Gain4 : Gain  Gain=-1i
  Gain5 : Gain  Gain=1i
  Gain6 : Gain  Gain=1/2
  Gain7 : Gain  Gain=1i
  NOT : Logic  Operator=NOT  IconShape=distinctive  AllPortsSameDT=off  OutDataTypeStr=boolean
  Product3 : Product
  Product4 : Product
  Real-Imag to Complex : RealImagToComplex
  Real-Imag to Complex1 : RealImagToComplex
  Sum1 : Sum  Inputs=|++
  Sum2 : Sum  Inputs=-+|
  Switch : Switch  Criteria=u2 ~= 0  SaturateOnIntegerOverflow=off  InputSameDT=off
  Terminator3 : Terminator
  Transport Delay2 : TransportDelay  DelayTime=1/4*(1/fg)  BufferSize=1024*4
  Transport Delay3 : TransportDelay  DelayTime=1/4*(1/fg)  BufferSize=1024*4
  abc to Alpha-Beta-Zero : spsabctoAlphaBetaZeroLib/abc to Alpha-Beta-Zero
  q+ : Outport
  d+ : Outport  Port=2
  q- : Outport  Port=3
  d- : Outport  Port=4
  wires:
  NOT/1 -> Switch/2
  Constant/1 -> NOT/1
  Switch/1 -> Product3/1
  Gain6/1 -> Switch/3
  Sum2/1 -> Gain1/1
  Transport Delay2/1 -> Real-Imag to Complex1/1
  Demux3/1 -> Real-Imag to Complex/1
  Complex to Real-Imag1/2 -> Transport Delay3/1
  Gain1/1 -> Product4/2
  Real-Imag to Complex/1 -> Complex to Real-Imag1/1, Sum2/2, Sum1/1, Switch/1
  Complex to Real-Imag3/1 -> d-/1
  Real-Imag to Complex1/1 -> Gain5/1
  Complex to Real-Imag1/1 -> Transport Delay2/1
  Transport Delay3/1 -> Real-Imag to Complex1/2
  Demux3/2 -> Real-Imag to Complex/2
  Product3/1 -> Complex to Real-Imag2/1
  Product4/1 -> Complex to Real-Imag3/1
  abc to Alpha-Beta-Zero/1 -> Demux3/1
  abc/1 -> abc to Alpha-Beta-Zero/1
  Exp3/1 -> Product4/1
  Complex to Real-Imag3/2 -> q-/1
  Complex to Real-Imag2/2 -> q+/1
  Demux3/3 -> Terminator3/1
  Sum1/1 -> Gain6/1
  Gain5/1 -> Sum2/1, Sum1/2
  Exp2/1 -> Product3/2
  Gain4/1 -> Exp2/1
  Theta/1 -> Gain4/1, Gain7/1
  Gain7/1 -> Exp3/1
  Complex to Real-Imag2/1 -> d+/1

== system power_13NodeTestFeeder_4VSC_PV_DEG_symmtrc_loads_/PV_Geno_GFL_VSC_at_634/PV-Geno with VSC_GFL_at_634     /VSC Control/Current Control ==
  theta_g : Inport
  w_g : Inport  Port=2
  V_qd : Inport  Port=3
  I_qd_ref : Inport  Port=4
  I_qd_c : Inport  Port=5
  Constant : Constant  Value=0
  Delay : Delay  DelayLength=1  InitialCondition=0.1
  Delay1 : Delay  DelayLength=1  InitialCondition=0.1
  Demux : Demux  Outputs=2
  Demux1 : Demux  Outputs=2
  Demux2 : Demux  Outputs=3
  Gain : Gain  Gain=Lc
  Inverse Park Transformation : Subsystem
  Mux : Mux  Inputs=3
  PID Controller : slpidlib/PID Controller  Controller=PI  Form=Parallel  TimeDomain=Continuous-time  UseExternalTs=off  SampleTime=-1  IntegratorMethod=Forward Euler  FilterMethod=Forward Euler  ControllerParametersSource=internal  P=Kp_C  I=Ki_C  UseKiTs=off  D=0  UseExternalDerivativeSource=off  N=100  UseFilter=on  TunerSelectOption=Transfer Function Based (PID Tuner App)  InitialConditionSource=internal  InitialConditionForIntegrator=0  InitialConditionForFilter=0  DifferentiatorICPrevScaledInput=0  ExternalReset=none  TrackingMode=off  Kt=1  LimitOutput=off  SatLimitsSource=internal  UpperSaturationLimit=inf  LowerSaturationLimit=-inf  LinearizeAsGain=on  AntiWindupMode=none  Kb=1  LimitIntegrator=off  UpperIntegratorSaturationLimit=inf  LowerIntegratorSaturationLimit=-inf  POutMin=[]  POutMax=[]  IOutMin=[]  IOutMax=[]  DOutMin=[]  DOutMax=[]  NOutMin=[]  NOutMax=[]  SumOutMin=[]  SumOutMax=[]  SaturationOutMin=[]  SaturationOutMax=[]  PParamMin=[]  PParamMax=[]  IParamMin=[]  IParamMax=[]  DParamMin=[]  DParamMax=[]  NParamMin=[]  NParamMax=[]  KbParamMin=[]  KbParamMax=[]  KtParamMin=[]  KtParamMax=[]  KbOutMin=[]  KbOutMax=[]  KtOutMin=[]  KtOutMax=[]  IntegratorOutMin=[]  IntegratorOutMax=[]  FilterOutMin=[]  FilterOutMax=[]  SumI1OutMin=[]  SumI1OutMax=[]  SumI2OutMin=[]  SumI2OutMax=[]  SumI3OutMin=[]  SumI3OutMax=[]  SumI4OutMin=[]  SumI4OutMax=[]  SumDOutMin=[]  SumDOutMax=[]  DifferentiatorOutMin=[]  DifferentiatorOutMax=[]  FilterDiffOutCoefMin=[]  FilterDiffOutCoefMax=[]  ReciprocalOutMin=[]  ReciprocalOutMax=[]  SumDenOutMin=[]  SumDenOutMax=[]  SumNumOutMin=[]  SumNumOutMax=[]  DivideOutMin=[]  DivideOutMax=[]  UdiffTsProdOutMin=[]  UdiffTsProdOutMax=[]  NTsProdOutMin=[]  NTsProdOutMax=[]  UintegralTsProdOutMin=[]  UintegralTsProdOutMax=[]  UngainTsProdOutMin=[]  UngainTsProdOutMax=[]  ClampingZeroOutDataTypeStr=Inherit: Inherit via back propagation  ClampingZeroOutMin=[]  ClampingZeroOutMax=[]  FilterDenConstantOutDataTypeStr=Inherit: Inherit via back propagation  FilterDenConstantOutMin=[]  FilterDenConstantOutMax=[]  PCopyOutDataTypeStr=Inherit: Inherit via back propagation  PCopyOutMin=[]  PCopyOutMax=[]  NCopyOutDataTypeStr=Inherit: Inherit via back propagation  NCopyOutMin=[]  NCopyOutMax=[]  IntegratorContinuousStateAttributes=''  IntegratorStateMustResolveToSignalObject=off  IntegratorRTWStateStorageClass=Auto  FilterContinuousStateAttributes=''  FilterStateMustResolveToSignalObject=off  FilterRTWStateStorageClass=Auto  ParallelPVariant=InternalParameters  IdealPVariant=Disabled  IVariant=InternalParameters  DVariant=Disabled  IntegratorVariant=Continuous  SatVariant=Disabled  AWVariant=Passthrough  PCopyVariant=Disabled  TRVariant=Disabled  FdbkBlocksVariant=Forward  IdealPFdbkVariant=Disabled  SatFdbkVariant=Disabled  DerivativeFilterVariant=Disabled  NVariant=Disabled  NCopyVariant=Disabled_SignalSpec  FilterICVariant=Disabled  IntegratorICVariant=InternalICs  ExternalResetVariant=Disabled  TRSumVariant=Passthrough  SumFdbkVariant=Disabled  SumVariant=Sum_PI  TsampFilterVariant=InternalTs  TsampNgainVariant=Passthrough  TsampIntegralVariant=Disabled_SignalSpec  ExternalSaturationOutDataTypeStr=Inherit: Same as second input  DerivativeSourceVariant=Disabled  PreIntVariant=InternalPreInt
  PID Controller1 : slpidlib/PID Controller  Controller=PI  Form=Parallel  TimeDomain=Continuous-time  UseExternalTs=off  SampleTime=-1  IntegratorMethod=Forward Euler  FilterMethod=Forward Euler  ControllerParametersSource=internal  P=Kp_C  I=Ki_C  UseKiTs=off  D=0  UseExternalDerivativeSource=off  N=100  UseFilter=on  TunerSelectOption=Transfer Function Based (PID Tuner App)  InitialConditionSource=internal  InitialConditionForIntegrator=0  InitialConditionForFilter=0  DifferentiatorICPrevScaledInput=0  ExternalReset=none  TrackingMode=off  Kt=1  LimitOutput=off  SatLimitsSource=internal  UpperSaturationLimit=inf  LowerSaturationLimit=-inf  LinearizeAsGain=on  AntiWindupMode=none  Kb=1  LimitIntegrator=off  UpperIntegratorSaturationLimit=inf  LowerIntegratorSaturationLimit=-inf  POutMin=[]  POutMax=[]  IOutMin=[]  IOutMax=[]  DOutMin=[]  DOutMax=[]  NOutMin=[]  NOutMax=[]  SumOutMin=[]  SumOutMax=[]  SaturationOutMin=[]  SaturationOutMax=[]  PParamMin=[]  PParamMax=[]  IParamMin=[]  IParamMax=[]  DParamMin=[]  DParamMax=[]  NParamMin=[]  NParamMax=[]  KbParamMin=[]  KbParamMax=[]  KtParamMin=[]  KtParamMax=[]  KbOutMin=[]  KbOutMax=[]  KtOutMin=[]  KtOutMax=[]  IntegratorOutMin=[]  IntegratorOutMax=[]  FilterOutMin=[]  FilterOutMax=[]  SumI1OutMin=[]  SumI1OutMax=[]  SumI2OutMin=[]  SumI2OutMax=[]  SumI3OutMin=[]  SumI3OutMax=[]  SumI4OutMin=[]  SumI4OutMax=[]  SumDOutMin=[]  SumDOutMax=[]  DifferentiatorOutMin=[]  DifferentiatorOutMax=[]  FilterDiffOutCoefMin=[]  FilterDiffOutCoefMax=[]  ReciprocalOutMin=[]  ReciprocalOutMax=[]  SumDenOutMin=[]  SumDenOutMax=[]  SumNumOutMin=[]  SumNumOutMax=[]  DivideOutMin=[]  DivideOutMax=[]  UdiffTsProdOutMin=[]  UdiffTsProdOutMax=[]  NTsProdOutMin=[]  NTsProdOutMax=[]  UintegralTsProdOutMin=[]  UintegralTsProdOutMax=[]  UngainTsProdOutMin=[]  UngainTsProdOutMax=[]  ClampingZeroOutDataTypeStr=Inherit: Inherit via back propagation  ClampingZeroOutMin=[]  ClampingZeroOutMax=[]  FilterDenConstantOutDataTypeStr=Inherit: Inherit via back propagation  FilterDenConstantOutMin=[]  FilterDenConstantOutMax=[]  PCopyOutDataTypeStr=Inherit: Inherit via back propagation  PCopyOutMin=[]  PCopyOutMax=[]  NCopyOutDataTypeStr=Inherit: Inherit via back propagation  NCopyOutMin=[]  NCopyOutMax=[]  IntegratorContinuousStateAttributes=''  IntegratorStateMustResolveToSignalObject=off  IntegratorRTWStateStorageClass=Auto  FilterContinuousStateAttributes=''  FilterStateMustResolveToSignalObject=off  FilterRTWStateStorageClass=Auto  ParallelPVariant=InternalParameters  IdealPVariant=Disabled  IVariant=InternalParameters  DVariant=Disabled  IntegratorVariant=Continuous  SatVariant=Disabled  AWVariant=Passthrough  PCopyVariant=Disabled  TRVariant=Disabled  FdbkBlocksVariant=Forward  IdealPFdbkVariant=Disabled  SatFdbkVariant=Disabled  DerivativeFilterVariant=Disabled  NVariant=Disabled  NCopyVariant=Disabled_SignalSpec  FilterICVariant=Disabled  IntegratorICVariant=InternalICs  ExternalResetVariant=Disabled  TRSumVariant=Passthrough  SumFdbkVariant=Disabled  SumVariant=Sum_PI  TsampFilterVariant=InternalTs  TsampNgainVariant=Passthrough  TsampIntegralVariant=Disabled_SignalSpec  ExternalSaturationOutDataTypeStr=Inherit: Same as second input  DerivativeSourceVariant=Disabled  PreIntVariant=InternalPreInt
  Product : Product
  Product1 : Product
  Sum : Sum  Inputs=|+-
  Sum1 : Sum  Inputs=-+|
  Sum2 : Sum  Inputs=+++
  Sum4 : Sum  Inputs=-++
  Terminator : Terminator
  V_abc_c : Outport
  wires:
  Demux2/2 -> Product1/2, Sum1/1
  V_qd/1 -> Demux/1
  Sum1/1 -> PID Controller1/1
  Sum/1 -> PID Controller/1
  Gain/1 -> Product/2, Product1/1
  Demux/2 -> [Vd]
  [Vd] -> Sum4/3
  Mux/1 -> Inverse Park Transformation/1(qd0)
  Constant/1 -> Mux/3
  Demux1/1 -> Sum/1
  Demux2/1 -> Sum/2, Product/1
  theta_g/1 -> Inverse Park Transformation/2(theta)
  Demux/1 -> [Vq]
  PID Controller/1 -> Sum2/2
  PID Controller1/1 -> Sum4/2
  Product1/1 -> Sum2/3
  [Vq] -> Sum2/1
  Inverse Park Transformation/1(abc) -> V_abc_c/1
  Product/1 -> Sum4/1
  Demux1/2 -> Sum1/2
  w_g/1 -> Gain/1
  I_qd_ref/1 -> Demux1/1
  I_qd_c/1 -> Demux2/1
  Demux2/3 -> Terminator/1
  Sum2/1 -> Delay/1
  Delay/1 -> Mux/1
  Delay1/1 -> Mux/2
  Sum4/1 -> Delay1/1
